simulink model "inverted_pendulum_digital_twin"  (R2022a)
settings: Solver=ode4  StartTime=0.0  StopTime=6.0  FixedStep=0.001  RelTol=1e-3
libraries: simulink x2
settings Model: Creator=Obay Zak  LastModifiedBy=Obay Zak

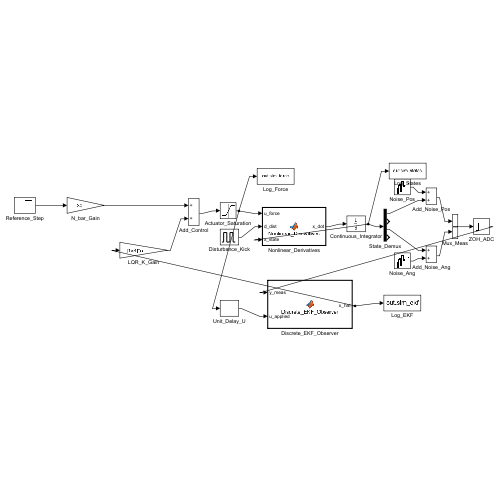
[thumbnail: Simulink's stored preview of the top-level diagram]
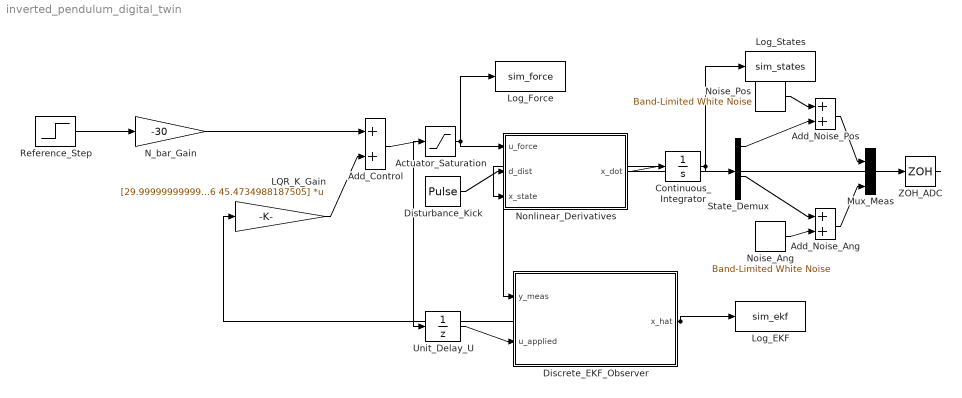
== system inverted_pendulum_digital_twin ==
  Actuator_Saturation : Saturate  UpperLimit=25.0  LowerLimit=-25.0
  Add_Control : Sum
  Add_Noise_Ang : Sum
  Add_Noise_Pos : Sum
  Continuous_Integrator : Integrator  InitialCondition=[0.0; 0.0; 0.087266; 0.0]
  Discrete_EKF_Observer : MATLAB Function  TreatAsAtomicUnit=on
  Disturbance_Kick : DiscretePulseGenerator  PulseType=Time based  Amplitude=0.0  Period=10.0  PulseWidth=1.0  PhaseDelay=3.0
  LQR_K_Gain : Gain  Gain=[29.9999999999999 41.3872908079915 317.147763700136 45.4734988187505]  Multiplication=Matrix(K*u)
  Log_EKF : ToWorkspace  VariableName=sim_ekf  SampleTime=0.005
  Log_Force : ToWorkspace  VariableName=sim_force  SampleTime=0.001
  Log_States : ToWorkspace  VariableName=sim_states  SampleTime=0.001
  Mux_Meas : Concatenate  ConcatenateDimension=2
  N_bar_Gain : Gain  Gain=-30
  Noise_Ang : simulink/Sources/Band-Limited White Noise  Cov=3.7e-5  Ts=0.005  seed=[23341]
  Noise_Pos : simulink/Sources/Band-Limited White Noise  Cov=2.5e-5  Ts=0.005  seed=[23341]
  Nonlinear_Derivatives : MATLAB Function  TreatAsAtomicUnit=on
  Reference_Step : Step  Time=1.0  Before=0.0  After=0.5  SampleTime=0.005
  State_Demux : Demux
  Unit_Delay_U : UnitDelay  InitialCondition=0.0  SampleTime=0.005  HasFrameUpgradeWarning=on
  ZOH_ADC : ZeroOrderHold  SampleTime=0.005
  wires:
  Reference_Step/1 -> N_bar_Gain/1
  N_bar_Gain/1 -> Add_Control/1
  LQR_K_Gain/1 -> Add_Control/2
  Add_Control/1 -> Actuator_Saturation/1
  Actuator_Saturation/1 -> Log_Force/1, Nonlinear_Derivatives/1(u_force), Unit_Delay_U/1
  Disturbance_Kick/1 -> Nonlinear_Derivatives/2(d_dist)
  Nonlinear_Derivatives/1(x_dot) -> Continuous_Integrator/1
  Continuous_Integrator/1 -> Nonlinear_Derivatives/3(x_state), State_Demux/1, Log_States/1
  Noise_Pos/1 -> Add_Noise_Pos/1
  State_Demux/1 -> Add_Noise_Pos/2
  Add_Noise_Pos/1 -> Mux_Meas/1
  State_Demux/3 -> Add_Noise_Ang/1
  Noise_Ang/1 -> Add_Noise_Ang/2
  Add_Noise_Ang/1 -> Mux_Meas/2
  Mux_Meas/1 -> ZOH_ADC/1
  ZOH_ADC/1 -> Discrete_EKF_Observer/1(y_meas)
  Unit_Delay_U/1 -> Discrete_EKF_Observer/2(u_applied)
  Discrete_EKF_Observer/1(x_hat) -> Log_EKF/1, LQR_K_Gain/1

== matlab function inverted_pendulum_digital_twin/Nonlinear_Derivatives ==
  data: u_force input; x_dot output; d_dist input; x_state input
function x_dot = Nonlinear_Derivatives(u_force, d_dist, x_state)
% Nominal physical parameters
M = 1.50; m = 0.25; l = 0.35; I = 0.010208; b = 0.10; c = 0.005; g = 9.81;

x_dot_val = x_state(2);
th        = x_state(3);
th_dot    = x_state(4);

F_total = u_force + d_dist;
sin_t = sin(th);
cos_t = cos(th);
D = (M + m)*(I + m*l^2) - (m*l*cos_t)^2;

term1 = F_total - b*x_dot_val + m*l*(th_dot^2)*sin_t;
term2 = m*g*l*sin_t - c*th_dot;

x_ddot  = ((I + m*l^2)*term1 - m*l*cos_t*term2) / D;
th_ddot = ((M + m)*term2 - m*l*cos_t*term1) / D;

x_dot = [x_dot_val; x_ddot; th_dot; th_ddot];
end

== matlab function inverted_pendulum_digital_twin/Discrete_EKF_Observer ==
  data: y_meas input; x_hat output; u_applied input
function x_hat = Discrete_EKF_Observer(y_meas, u_applied)
persistent x_est P_cov;
Ts = 0.005;
if isempty(x_est)
    x_est = [0.0; 0.0; 0.0; 0.0];
    P_cov = diag([0.01, 0.1, 0.005, 0.05]);
end
M = 1.50; m = 0.25; l = 0.35; I = 0.010208; b = 0.10; c = 0.005; g = 9.81;
Q_d = diag([1e-6, 1e-4, 7.6e-7, 7.6e-5]);
R_d = diag([2.5e-5, 3.7e-5]);

% 1. State Prediction
x_dot = [x_est(2);
         (-(I+m*l^2)*b*x_est(2) + m^2*g*l^2*x_est(3) - m*l*c*x_est(4) + (I+m*l^2)*u_applied) / 0.063802;
         x_est(4);
         (m*l*b*x_est(2) + (M+m)*m*g*l*x_est(3) - (M+m)*c*x_est(4) - m*l*u_applied) / 0.063802];
x_pred = x_est + Ts * x_dot;

% 2. System Jacobian Phi
F_mat = [0, 1, 0, 0;
         0, -0.0640, 1.1771, -0.0069;
         0, 0, 0, 1;
         0, 0.1371, 23.5440, -0.1371];
Phi = eye(4) + F_mat * Ts;
P_pred = Phi * P_cov * Phi' + Q_d;

% 3. Measurement Update
H = [1, 0, 0, 0; 0, 0, 1, 0];
S = H * P_pred * H' + R_d;
K = (P_pred * H') / S;
y_res = y_meas - H * x_pred;
x_est = x_pred + K * y_res;
I_KH = eye(4) - K * H;
P_cov = I_KH * P_pred * I_KH' + K * R_d * K';
x_hat = x_est;
end
